simulink model "snap"  (R2023a)
settings: Solver=VariableStepAuto  StartTime=0.0  StopTime=80  RelTol=1e-3
libraries: shareduavrstlib x1, simulink x1
settings Model: Creator=zhiyu  LastModifiedBy=zhiyu

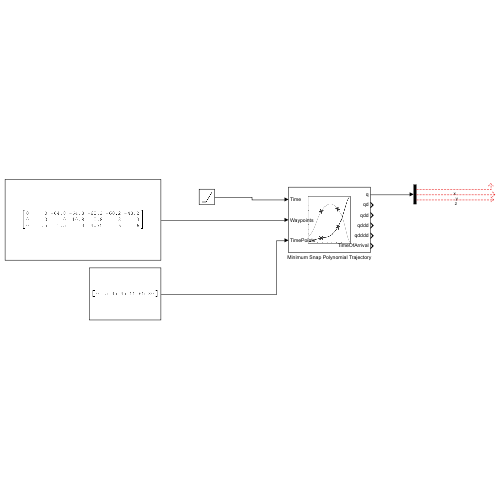
[thumbnail: Simulink's stored preview of the top-level diagram]
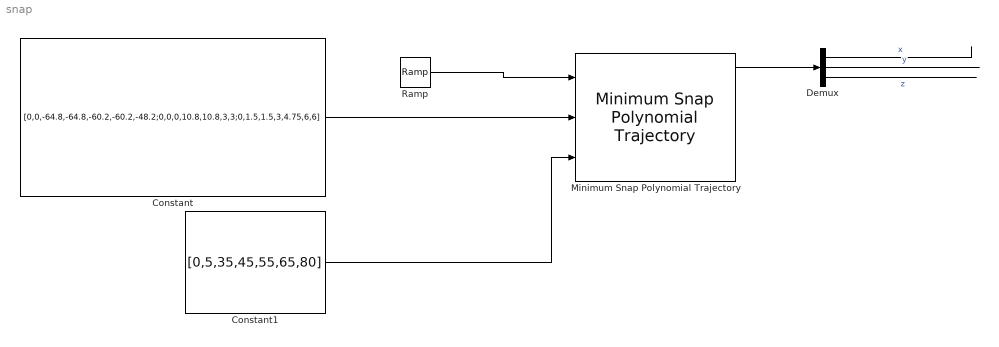
== system snap ==
  Constant : Constant  Value=[0,0,-64.8,-64.8,-60.2,-60.2,-48.2;0,0,0,10.8,10.8,3,3;0,1.5,1.5,3,4.75,6,6]  VectorParams1D=off
  Constant1 : Constant  Value=[0,5,35,45,55,65,80]  VectorParams1D=off
  Demux : Demux  Outputs=3
  Minimum Snap Polynomial Trajectory : shareduavrstlib/Minimum Snap Polynomial Trajectory  ShowBCInputPort=off  ShowPolynomialCoefs=off  ShowStatusOutputPort=off  TimeAllocation=off  TimeWeight=100  MinSegmentTime=0.1  MaxSegmentTime=1  MaxIteration=1500  MaxTime=10  SimulateUsing=Interpreted execution
      settings: LibrarySourceBlock=robotutilslib/Minimum Snap Polynomial Trajectory
  Ramp : simulink/Sources/Ramp  slope=1  start=0  InitialOutput=0
  wires:
  Minimum Snap Polynomial Trajectory/1 -> Demux/1
  Demux/1 -> ?  "x"
  Demux/2 -> ?  "y"
  Demux/3 -> ?  "z"
  Constant/1 -> Minimum Snap Polynomial Trajectory/2
  Ramp/1 -> Minimum Snap Polynomial Trajectory/1
  Constant1/1 -> Minimum Snap Polynomial Trajectory/3
